simulink model "etc_PI"  (Simulink 10.1)
settings: Solver=ode45  StartTime=0.0  StopTime=20.0  RelTol=1e-3  EnableMultiTasking=on
model workspace (MAT data in the model file):
  Ki = 2
  Kp = 0.3
  Ts : num (value not decoded)
settings Model: Creator=cjz  LastModifiedBy=wkmia
settings DataIOCC: LimitDataPoints=on  SignalLoggingSaveFormat=ModelDataLogs
settings OptimizationCC: ExpressionDepthLimit=2147483647
settings DebuggingCC: SolverPrmCheckMsg=warning  FcnCallInpInsideContextMsg=warning  StateNameClashWarn=warning

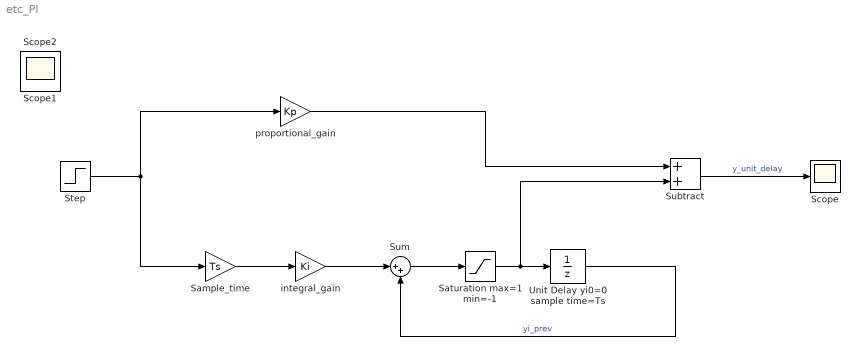
== system etc_PI ==
  Sample_time : Gain  Gain=Ts
  Saturation max=1 min=-1 : Saturate  UpperLimit=1  LowerLimit=-1
  Scope : Scope
  Step : Step  SampleTime=0
  Subtract : Sum
  Sum : Sum  Inputs=|++
  Unit Delay yi0=0 sample time=Ts : UnitDelay  SampleTime=Ts
  integral_gain : Gain  Gain=Ki
  proportional_gain : Gain  Gain=Kp
  Scope1 : Scope
  Scope2 : Scope
  wires:
  proportional_gain/1 -> Subtract/1
  Unit Delay yi0=0 sample time=Ts/1 -> Sum/2  "yi_prev"
  Sum/1 -> Saturation max=1 min=-1/1
  Saturation max=1 min=-1/1 -> Unit Delay yi0=0 sample time=Ts/1, Subtract/2
  Sample_time/1 -> integral_gain/1
  integral_gain/1 -> Sum/1
  Subtract/1 -> Scope/1  "y_unit_delay"
  Step/1 -> Sample_time/1, proportional_gain/1
